simulink model "Tracer_New_Version"  (R2025a)
settings: Solver=FixedStepAuto  StartTime=0.0  StopTime=inf  RelTol=1e-3  EnableMultiTasking=on
undefined symbols (not defined in the file): bits
libraries: stm32blockslib x30, stm32f4xxblockslib x10, svdutilitieslib x10, simulink x5
(part 2 of 2)

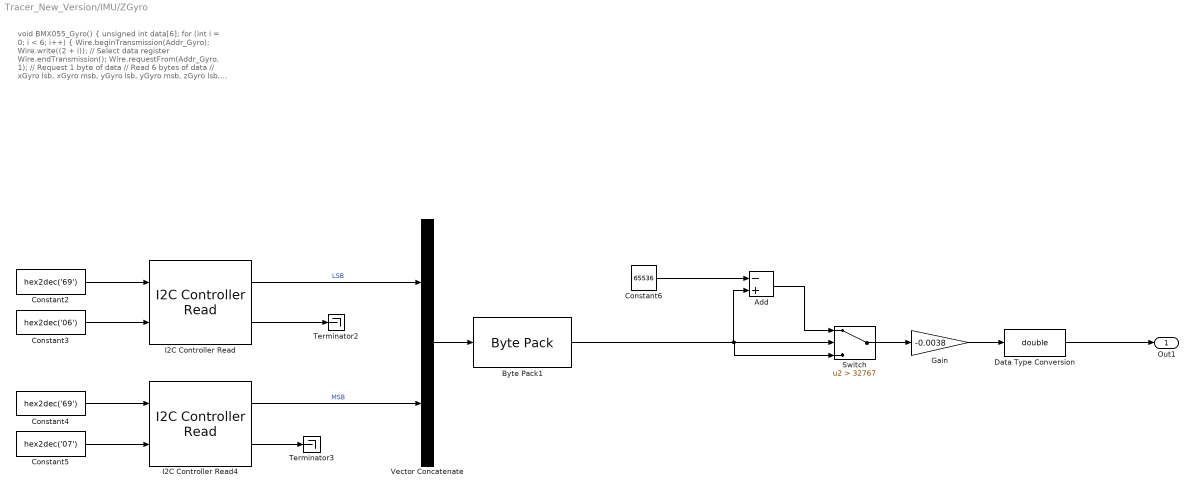
== system Tracer_New_Version/IMU/ZGyro ==
  note: void BMX055_Gyro()
      | {
      | unsigned int data[6];
      | for (int i = 0; i < 6; i++)
      | {
      | Wire.beginTransmission(Addr_Gyro);
      | Wire.write((2 + i)); // Select data register
      | Wire.endTransmission();
      | Wire.requestFrom(Addr_Gyro, 1); // Request 1 byte of data
      | // Read 6 bytes of data
      | // xGyro lsb, xGyro msb, yGyro lsb, yGyro msb, zGyro lsb, zGyro msb
      | if (Wire.available() == 1)
      | data[i] = Wire.read();
      | }
      | // Convert the data
      | zGyro = (data[5] * 256) + data[4];
      | if (zGyro > 32767) zGyro -= 65536;
      | zGyro = zGyro * 0.0038; // Full scale = +/- 125 degree/s
      | }
  Add : Sum  Inputs=-+
  Byte Pack1 : svdutilitieslib/Byte Pack  maskPackedDataType=uint16  datatypes={'uint8'}  byteAlign=1  blockPlatform=arduinoert
      settings: LibrarySourceBlock=mcblib/Signal Management/Byte Pack
  Constant2 : Constant  Value=hex2dec('69')  OutDataTypeStr=uint8
  Constant3 : Constant  Value=hex2dec('06')  OutDataTypeStr=uint8
  Constant4 : Constant  Value=hex2dec('69')  OutDataTypeStr=uint8
  Constant5 : Constant  Value=hex2dec('07')  OutDataTypeStr=uint8
  Constant6 : Constant  Value=65536
  Data Type Conversion : DataTypeConversion  OutDataTypeStr=double  SaturateOnIntegerOverflow=off  RndMeth=Floor
  Gain : Gain  Gain=-0.0038
  I2C Controller Read : stm32blockslib/I2C Controller Read  I2CModule=I2C1  Mode=Controller  AddressingMode=7-bits  PeripheralByteOrder=LittleEndian  OwnPeripheralAddress=uint8(170)  PeripheralAddressVia=Inport  PeripheralAddress=0x19  RegisterAddressMode=on  RegisterAddressVia=Inport  RegisterAddress=0x02  RepeatedStart=off  NoAck=off  OutputStatus=on  BlockMode=Receive  DataType=uint8  DataLength=1  Timeout=0.001  SampleTime=-1
      settings: LibrarySourceBlock=stm32f4xxblockslib/I2C Controller Read
  I2C Controller Read4 : stm32blockslib/I2C Controller Read  I2CModule=I2C1  Mode=Controller  AddressingMode=7-bits  PeripheralByteOrder=LittleEndian  OwnPeripheralAddress=uint8(170)  PeripheralAddressVia=Inport  PeripheralAddress=0x19  RegisterAddressMode=on  RegisterAddressVia=Inport  RegisterAddress=0x02  RepeatedStart=off  NoAck=off  OutputStatus=on  BlockMode=Receive  DataType=uint8  DataLength=1  Timeout=0.001  SampleTime=-1
      settings: LibrarySourceBlock=stm32f4xxblockslib/I2C Controller Read
  Switch : Switch  Criteria=u2 > Threshold  Threshold=32767  SaturateOnIntegerOverflow=off  InputSameDT=off
  Terminator2 : Terminator
  Terminator3 : Terminator
  Vector Concatenate : Concatenate
  Out1 : Outport
  wires:
  Constant3/1 -> I2C Controller Read/2
  Add/1 -> Switch/1
  Constant4/1 -> I2C Controller Read4/1
  Gain/1 -> Data Type Conversion/1
  I2C Controller Read/2 -> Terminator2/1
  Constant2/1 -> I2C Controller Read/1
  Byte Pack1/1 -> Switch/2, Switch/3, Add/2
  Constant6/1 -> Add/1
  I2C Controller Read4/2 -> Terminator3/1
  I2C Controller Read4/1 -> Vector Concatenate/2  "MSB"
  Constant5/1 -> I2C Controller Read4/2
  Switch/1 -> Gain/1
  I2C Controller Read/1 -> Vector Concatenate/1  "LSB"
  Vector Concatenate/1 -> Byte Pack1/1
  Data Type Conversion/1 -> Out1/1
